simulink model "sampleModel2074"  (R2023a)
settings: Solver=VariableStepAuto  StartTime=0.0  StopTime=10.0  RelTol=1e-3
libraries: hdlsllib x6, simulink x1
settings Model: Creator=user1  LastModifiedBy=user1

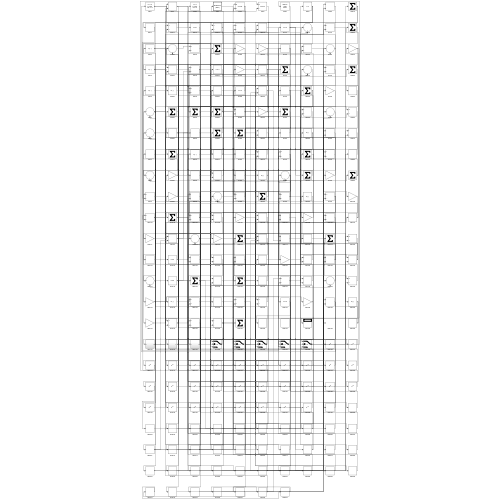
[thumbnail: Simulink's stored preview of the top-level diagram]
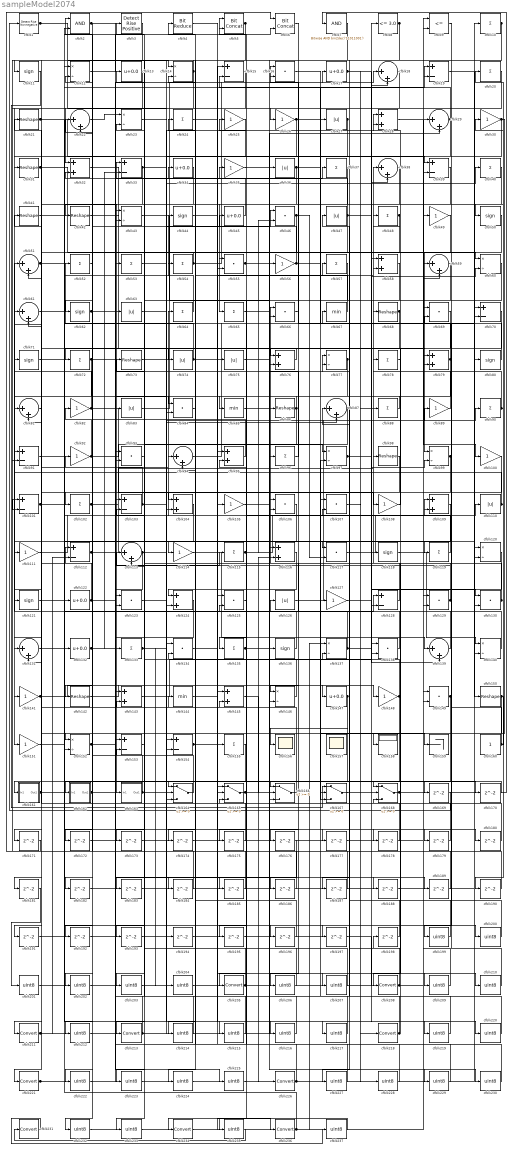
== system sampleModel2074 ==
  cfblk1 : hdlsllib/Logic and Bit Operations/Detect Rise Nonnegative  vinit=0  OutDataTypeStr=boolean
  cfblk{10,20,24,37,40,48,52..54,57,64..65,72,78,88,90,96,102,115,119,133,135,155} (23 alike) : Sum  Inputs=+
  cfblk{25..26,30,35,49,56,82,89,92,100,105,108,111,114,127,141,148,151} (18 alike) : Gain
  cfblk{15,19,33,39,70,91,101,103,112,128,153..154} (12 alike) : Sum  Inputs=+-
  cfblk{28,32,58,76,79,95,104,109,116,124,143,145} (12 alike) : Sum
  cfblk{16,46,55,66,69,84,93,106..107,117,123,125,129..130,134,138,149} (17 alike) : DotProduct  OutDataTypeStr=Inherit: Inherit via internal rule
  cfblk{11,44,50,62,71,80,118,121,136} (9 alike) : Signum
  cfblk{27,36,47,63,74..75,83,110,126} (9 alike) : Abs  SaturateOnIntegerOverflow=off
  cfblk{18,22,29,38,51,59,61,81,87,94,113,131,139} (13 alike) : Sum  Inputs=|++
  cfblk{12,14,23,43,60,77,97,99,120,137,140,146,152} (13 alike) : Product  Inputs=*/  RndMeth=Zero  SaturateOnIntegerOverflow=on
  cfblk{13,17,34,45,122,132,147} (7 alike) : Bias  Bias=0.0  SaturateOnIntegerOverflow=off
  cfblk{21,31,41..42,68,73,86,98,142,150} (10 alike) : Reshape
  cfblk144 : MinMax
  cfblk156 : Scope
  cfblk157 : Scope
      settings: Floating=on
  cfblk158 : Display
  cfblk159 : Terminator
  cfblk160 : Constant  SampleTime=-1
  cfblk161 : Subsystem
      settings: LibrarySourceBlock=|
      | hdlsllib/Ports &
      | Subsystems/Subsystem
  cfblk162 : Subsystem
      settings: LibrarySourceBlock=|
      | hdlsllib/Ports &
      | Subsystems/Subsystem
  cfblk163 : Subsystem
      settings: LibrarySourceBlock=|
      | hdlsllib/Ports &
      | Subsystems/Subsystem
  cfblk{164..168} (5 alike) : Switch  SaturateOnIntegerOverflow=off  InputSameDT=off
  cfblk{169..198} (30 alike) : Delay  SampleTime=1
  cfblk{199..204,206..207,209..210,212,214..217,219..220,222..225,227..230,232..233,235,237} (29 alike) : DataTypeConversion  OutDataTypeStr=uint8  SaturateOnIntegerOverflow=off  RndMeth=Floor
  cfblk2 : Logic  AllPortsSameDT=off  OutDataTypeStr=boolean
  cfblk{205,208,211,213,218,221,226,231,234,236} (10 alike) : DataTypeConversion  SaturateOnIntegerOverflow=off  RndMeth=Floor
  cfblk3 : hdlsllib/Logic and Bit Operations/Detect Rise Positive  vinit=0  OutDataTypeStr=boolean
  cfblk4 : hdlsllib/Logic and Bit Operations/Bit Reduce  mode=AND
  cfblk5 : hdlsllib/Logic and Bit Operations/Bit Concat  numInputs=2
  cfblk6 : hdlsllib/Logic and Bit Operations/Bit Concat  numInputs=2
  cfblk67 : MinMax
  cfblk7 : simulink/Logic and Bit Operations/Bitwise Operator  logicop=AND  UseBitMask=on  BitMask=bin2dec('11011001')  BitMaskRealWorld=Stored Integer
      settings: LibrarySourceBlock=|
      | hdlsllib/Logic and Bit
      | Operations/Bitwise
      | Operator
  cfblk8 : hdlsllib/Logic and Bit Operations/Compare To Constant  relop=<=  const=3.0  OutDataTypeStr=boolean
  cfblk85 : MinMax
  cfblk9 : RelationalOperator  Operator=<=  OutDataTypeStr=boolean  InputSameDT=off
  wires:
  cfblk118/1 -> cfblk140/1
  cfblk72/1 -> cfblk151/1, cfblk177/1
  cfblk50/1 -> cfblk102/1
  cfblk54/1 -> cfblk18/1, cfblk53/1, cfblk117/1
  cfblk25/1 -> cfblk141/1
  cfblk110/1 -> cfblk50/1, cfblk91/1
  cfblk74/1 -> cfblk52/1, cfblk178/1
  cfblk33/1 -> cfblk163/1(In1), cfblk188/1
  cfblk139/1 -> cfblk51/1
  cfblk30/1 -> cfblk158/1, cfblk104/2
  cfblk36/1 -> cfblk65/1, cfblk138/2, cfblk124/2, cfblk120/2
  cfblk129/1 -> cfblk38/1, cfblk113/1
  cfblk146/1 -> cfblk5/1
  cfblk13/1 -> cfblk31/1
  cfblk57/1 -> cfblk135/1
  cfblk40/1 -> cfblk111/1
  cfblk134/1 -> cfblk57/1
  cfblk83/1 -> cfblk17/1
  cfblk31/1 -> cfblk99/1, cfblk79/2
  cfblk88/1 -> cfblk81/1
  cfblk111/1 -> cfblk64/1
  cfblk128/1 -> cfblk66/1
  cfblk43/1 -> cfblk96/1
  cfblk90/1 -> cfblk30/1, cfblk78/1
  cfblk125/1 -> cfblk205/1
  cfblk19/1 -> cfblk150/1
  cfblk5/1 -> cfblk84/1, cfblk203/1
  cfblk29/1 -> cfblk15/2, cfblk171/1
  cfblk130/1 -> cfblk45/1, cfblk33/1
  cfblk112/1 -> cfblk94/1, cfblk63/1
  cfblk39/1 -> cfblk76/1
  cfblk73/1 -> cfblk10/1
  cfblk65/1 -> cfblk86/1
  cfblk37/1 -> cfblk62/1
  cfblk107/1 -> cfblk218/1
  cfblk2/1 -> cfblk167/2, cfblk84/2, cfblk222/1
  cfblk135/1 -> cfblk136/1, cfblk58/2
  cfblk136/1 -> cfblk126/1
  cfblk64/1 -> cfblk44/1
  cfblk116/1 -> cfblk124/1
  cfblk17/1 -> cfblk130/1, cfblk88/1, cfblk228/1
  cfblk87/1 -> cfblk195/1, cfblk214/1
  cfblk114/1 -> cfblk139/1
  cfblk133/1 -> cfblk87/2, cfblk204/1
  cfblk126/1 -> cfblk90/1
  cfblk98/1 -> cfblk121/1
  cfblk10/1 -> cfblk91/2, cfblk206/1
  cfblk94/1 -> cfblk27/1
  cfblk41/1 -> cfblk122/1
  cfblk152/1 -> cfblk92/1, cfblk115/1
  cfblk14/1 -> cfblk32/1, cfblk11/1
  cfblk138/1 -> cfblk13/1
  cfblk137/1 -> cfblk110/1, cfblk112/1
  cfblk22/1 -> cfblk23/1
  cfblk115/1 -> cfblk18/2, cfblk46/2
  cfblk62/1 -> cfblk16/2, cfblk225/1
  cfblk26/1 -> cfblk60/1, cfblk43/2
  cfblk119/1 -> cfblk25/1
  cfblk121/1 -> cfblk6/2
  cfblk141/1 -> cfblk147/1, cfblk196/1
  cfblk95/1 -> cfblk2/1
  cfblk69/1 -> cfblk208/1
  cfblk150/1 -> cfblk190/1, cfblk191/1
  cfblk102/1 -> cfblk98/1, cfblk215/1
  cfblk155/1 -> cfblk211/1
  cfblk92/1 -> cfblk97/1, cfblk82/1
  cfblk8/1 -> cfblk42/1, cfblk164/3, cfblk187/1
  cfblk145/1 -> cfblk226/1
  cfblk15/1 -> cfblk152/1
  cfblk82/1 -> cfblk108/1, cfblk41/1
  cfblk80/1 -> cfblk68/1
  cfblk70/1 -> cfblk221/1
  cfblk27/1 -> cfblk104/1, cfblk172/1
  cfblk67/1 -> cfblk24/1
  cfblk78/1 -> cfblk168/1
  cfblk108/1 -> cfblk28/1
  cfblk132/1 -> cfblk33/2, cfblk180/1, cfblk189/1
  cfblk147/1 -> cfblk156/1, cfblk165/2
  cfblk20/1 -> cfblk26/1
  cfblk113/1 -> cfblk123/1, cfblk186/1
  cfblk81/1 -> cfblk131/1
  cfblk45/1 -> cfblk4/1
  cfblk104/1 -> cfblk131/2
  cfblk56/1 -> cfblk19/1, cfblk12/2
  cfblk161/1(Out1) -> cfblk109/1, cfblk219/1
  cfblk153/1 -> cfblk213/1
  cfblk51/1 -> cfblk132/1, cfblk19/2
  cfblk6/1 -> cfblk146/1
  cfblk21/1 -> cfblk83/1, cfblk43/1
  cfblk154/1 -> cfblk105/1, cfblk197/1
  cfblk127/1 -> cfblk38/2
  cfblk84/1 -> cfblk34/1
  cfblk55/1 -> cfblk56/1, cfblk230/1
  cfblk123/1 -> cfblk46/1
  cfblk61/1 -> cfblk119/1
  cfblk11/1 -> cfblk167/1
  cfblk142/1 -> cfblk148/1
  cfblk143/1 -> cfblk8/1
  cfblk47/1 -> cfblk22/2, cfblk139/2, cfblk81/2, cfblk133/1, cfblk232/1
  cfblk162/1(Out1) -> cfblk37/1, cfblk184/1
  cfblk75/1 -> cfblk79/1
  cfblk58/1 -> cfblk103/1
  cfblk96/1 -> cfblk76/2
  cfblk16/1 -> cfblk159/1
  cfblk18/1 -> cfblk101/2
  cfblk151/1 -> cfblk128/1
  cfblk109/1 -> cfblk152/2
  cfblk166/1 -> cfblk21/1
  cfblk38/1 -> cfblk142/1
  cfblk68/1 -> cfblk162/1(In1), cfblk167/3
  cfblk63/1 -> cfblk28/2
  cfblk149/1 -> cfblk164/2, cfblk212/1
  cfblk99/1 -> cfblk174/1, cfblk175/1
  cfblk101/1 -> cfblk114/1, cfblk67/1
  cfblk1/1 -> cfblk14/1, cfblk154/2
  cfblk23/1 -> cfblk39/1
  cfblk77/1 -> cfblk94/2, cfblk173/1
  cfblk140/1 -> cfblk116/1
  cfblk89/1 -> cfblk48/1
  cfblk120/1 -> cfblk128/2
  cfblk42/1 -> cfblk127/1
  cfblk167/1 -> cfblk60/2
  cfblk4/1 -> cfblk95/1
  cfblk48/1 -> cfblk123/2, cfblk227/1
  cfblk86/1 -> cfblk85/1, cfblk233/1
  cfblk46/1 -> cfblk66/2, cfblk117/2
  cfblk163/1(Out1) -> cfblk22/1, cfblk89/1
  cfblk91/1 -> cfblk54/1
  cfblk122/1 -> cfblk77/1, cfblk71/1
  cfblk103/1 -> cfblk40/1, cfblk61/1
  cfblk76/1 -> cfblk74/1
  cfblk148/1 -> cfblk3/1, cfblk182/1
  cfblk32/1 -> cfblk55/1
  cfblk24/1 -> cfblk75/1
  cfblk34/1 -> cfblk161/1(In1)
  cfblk164/1 -> cfblk23/2
  cfblk97/1 -> cfblk77/2, cfblk99/2
  cfblk160/1 -> cfblk20/1, cfblk109/2
  cfblk168/1 -> cfblk7/1, cfblk120/1
  cfblk79/1 -> cfblk16/1, cfblk192/1
  cfblk100/1 -> cfblk164/1
  cfblk12/1 -> cfblk5/2
  cfblk28/1 -> cfblk100/1
  cfblk52/1 -> cfblk72/1
  cfblk117/1 -> cfblk80/1
  cfblk165/1 -> cfblk29/2, cfblk116/2, cfblk209/1
  cfblk7/1 -> cfblk166/3
  cfblk131/1 -> cfblk169/1
  cfblk169/1 -> cfblk1/1
  cfblk44/1 -> cfblk170/1
  cfblk170/1 -> cfblk166/1
  cfblk171/1 -> cfblk6/1
  cfblk172/1 -> cfblk55/2
  cfblk173/1 -> cfblk97/2
  cfblk174/1 -> cfblk29/1
  cfblk175/1 -> cfblk61/2
  cfblk66/1 -> cfblk176/1
  cfblk177/1 -> cfblk39/2
  cfblk178/1 -> cfblk95/2
  cfblk71/1 -> cfblk179/1
  cfblk179/1 -> cfblk15/1
  cfblk180/1 -> cfblk51/2
  cfblk3/1 -> cfblk181/1
  cfblk182/1 -> cfblk130/2
  cfblk124/1 -> cfblk183/1
  cfblk183/1 -> cfblk149/2
  cfblk184/1 -> cfblk113/2
  cfblk60/1 -> cfblk185/1
  cfblk185/1 -> cfblk101/1
  cfblk186/1 -> cfblk32/2
  cfblk187/1 -> cfblk103/2
  cfblk188/1 -> cfblk168/3
  cfblk189/1 -> cfblk165/3
  cfblk190/1 -> cfblk166/2
  cfblk191/1 -> cfblk2/2
  cfblk192/1 -> cfblk146/2
  cfblk93/1 -> cfblk193/1
  cfblk193/1 -> cfblk134/1
  cfblk195/1 -> cfblk168/2
  cfblk196/1 -> cfblk14/2
  cfblk198/1 -> cfblk137/2
  cfblk9/1 -> cfblk199/1
  cfblk199/1 -> cfblk47/1
  cfblk85/1 -> cfblk200/1
  cfblk200/1 -> cfblk9/1
  cfblk181/1 -> cfblk201/1
  cfblk201/1 -> cfblk9/2
  cfblk106/1 -> cfblk202/1
  cfblk202/1 -> cfblk58/1
  cfblk203/1 -> cfblk106/1
  cfblk204/1 -> cfblk106/2
  cfblk205/1 -> cfblk143/2, cfblk138/1
  cfblk206/1 -> cfblk125/1
  cfblk105/1 -> cfblk207/1
  cfblk207/1 -> cfblk125/2
  cfblk208/1 -> cfblk118/1, cfblk87/1
  cfblk209/1 -> cfblk69/1
  cfblk194/1 -> cfblk210/1
  cfblk210/1 -> cfblk69/2
  cfblk211/1 -> cfblk165/1, cfblk112/2, cfblk36/1
  cfblk212/1 -> cfblk155/1
  cfblk213/1 -> cfblk194/1, cfblk93/1
  cfblk214/1 -> cfblk153/1
  cfblk215/1 -> cfblk153/2
  cfblk144/1 -> cfblk216/1
  cfblk216/1 -> cfblk154/1
  cfblk53/1 -> cfblk217/1
  cfblk217/1 -> cfblk144/1
  cfblk218/1 -> cfblk198/1, cfblk73/1
  cfblk219/1 -> cfblk107/1
  cfblk197/1 -> cfblk220/1
  cfblk220/1 -> cfblk107/2
  cfblk221/1 -> cfblk93/2, cfblk149/1
  cfblk222/1 -> cfblk70/1
  cfblk176/1 -> cfblk223/1
  cfblk223/1 -> cfblk70/2
  cfblk49/1 -> cfblk224/1
  cfblk224/1 -> cfblk140/2
  cfblk225/1 -> cfblk49/1
  cfblk226/1 -> cfblk143/1, cfblk129/1
  cfblk227/1 -> cfblk145/1
  cfblk228/1 -> cfblk145/2
  cfblk35/1 -> cfblk229/1
  cfblk229/1 -> cfblk134/2
  cfblk230/1 -> cfblk35/1
  cfblk232/1 -> cfblk59/1
  cfblk233/1 -> cfblk59/2
  cfblk234/1 -> cfblk236/1
  cfblk59/1 -> cfblk235/1
  cfblk235/1 -> cfblk231/1
  cfblk236/1 -> cfblk12/1, cfblk129/2, cfblk137/1
  cfblk231/1 -> cfblk237/1
  cfblk237/1 -> cfblk234/1

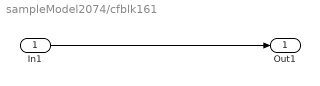
== system sampleModel2074/cfblk161 ==
  In1 : Inport
  Out1 : Outport
  wires:
  In1/1 -> Out1/1

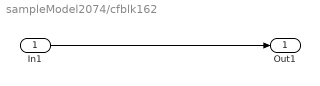
== system sampleModel2074/cfblk162 ==
  In1 : Inport
  Out1 : Outport
  wires:
  In1/1 -> Out1/1

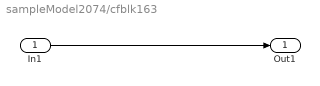
== system sampleModel2074/cfblk163 ==
  In1 : Inport
  Out1 : Outport
  wires:
  In1/1 -> Out1/1
